simulink model "RelayH"  (R2020a)
settings: Solver=FixedStepAuto  StartTime=0.0  StopTime=100  RelTol=1e-3
undefined symbols (not defined in the file or in its folder): delay, epsilon, G_dem, G_num, Ra
settings Model: Creator=jlula  LastModifiedBy=João Lula
settings SFSimCC: CustomCodeUndefinedFunction=UseInterfaceOnly

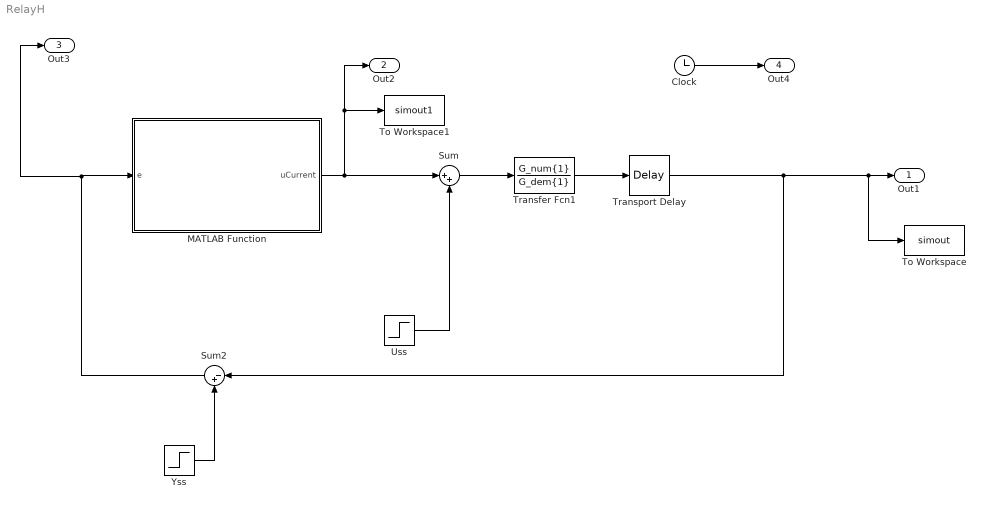
== system RelayH ==
  Clock : Clock
  MATLAB Function : MATLAB Function  TreatAsAtomicUnit=on
  Sum : Sum  Inputs=|++
  Sum2 : Sum  Inputs=|-+
  To Workspace : ToWorkspace  VariableName=simout  SaveFormat=Timeseries  SampleTime=-1
  To Workspace1 : ToWorkspace  VariableName=simout1  SaveFormat=Timeseries  SampleTime=-1
  Transfer Fcn1 : TransferFcn  Numerator=G_num{1}  Denominator=G_dem{1}
  Transport Delay : TransportDelay  DelayTime=delay
  Uss : Step  Time=0  Before=150  After=150  SampleTime=0
  "Yss " : Step  Time=0  After=150  SampleTime=0
  Out1 : Outport  SignalName=y  VectorParamsAs1DForOutWhenUnconnected=off
  Out2 : Outport  Port=2  SignalName=u  VectorParamsAs1DForOutWhenUnconnected=off
  Out3 : Outport  Port=3  SignalName=e  VectorParamsAs1DForOutWhenUnconnected=off
  Out4 : Outport  Port=4  SignalName=t  VectorParamsAs1DForOutWhenUnconnected=off
  wires:
  MATLAB Function/1(uCurrent) -> To Workspace1/1, Out2/1, Sum/1
  Uss/1 -> Sum/2
  Transport Delay/1 -> To Workspace/1, Out1/1, Sum2/1
  "Yss "/1 -> Sum2/2
  Sum2/1 -> Out3/1, MATLAB Function/1(e)
  Clock/1 -> Out4/1
  Sum/1 -> Transfer Fcn1/1
  Transfer Fcn1/1 -> Transport Delay/1

== matlab function RelayH/MATLAB Function ==
  settings: updateMethod=DISCRETE  sampleTime=Deltat
  data: e input; uCurrent output; Ra parameter; epsilon parameter
function uCurrent = RelayH(e, Ra, epsilon)
   

    persistent uPast
    if isempty(uPast)
        uPast=Ra;
    end
    if abs(e)<=epsilon
        uCurrent=uPast;
    else
        uCurrent=sign(e)*Ra;
        uPast=uCurrent;
    end
end
